simulink model "ver1_mck_system"  (R2019a)
settings: Solver=FixedStepAuto  StartTime=0.0  StopTime=30  FixedStep=10e-5  RelTol=1e-3
InitFcn:
  | ver1_mck_system_m
values from neighbouring files (symbols this model uses):
  C = [1,0 ... (first row only)    [ver1_mck_system_m.m]    (also in ver2_vanderpol_system_m.m)
  dt = 0.001    [ver1_mck_system_m.m]    (also in ver2_vanderpol_system_m.m)
  general_constants = [m ... (first row only)    [ver1_mck_system_m.m]    (also in ver2_vanderpol_system_m.m = [mu])
  H = [1, 0 ... (first row only)    [ver1_mck_system_m.m]    (also in ver2_vanderpol_system_m.m)
  init_cond_cont = [0 ... (first row only)    [ver1_mck_system_m.m]    (also in ver2_vanderpol_system_m.m = [2)
  init_cond_disc = init_cond_cont    [ver1_mck_system_m.m]    (also in ver2_vanderpol_system_m.m)
  MNV = MNstd*MNstd    (= 0.0016)    [ver1_mck_system_m.m]    (also in ver2_vanderpol_system_m.m)
  P_init_disc = MNV*eye(2)    [ver1_mck_system_m.m]    (also in ver2_vanderpol_system_m.m)
  Q = 0*eye(2)*PNV    [ver1_mck_system_m.m]    (also in ver2_vanderpol_system_m.m = 0.2*eye(2)*PNV)
  R = 0.001*eye(2)*MNV    [ver1_mck_system_m.m]    (also in ver2_vanderpol_system_m.m = 60*eye(2)*MNV)
settings Model: Creator=Mehmet  LastModifiedBy=Mehmet

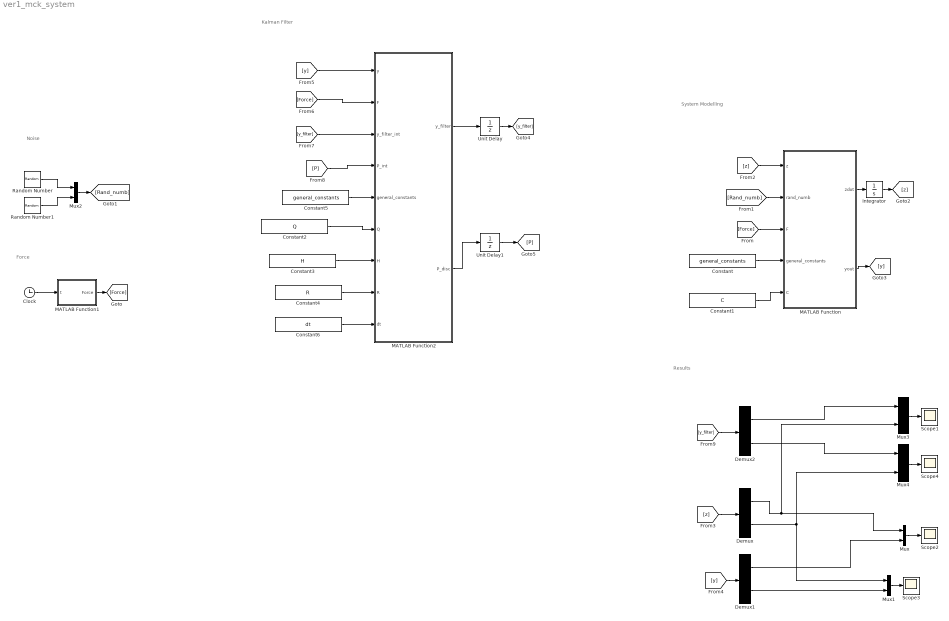
== system ver1_mck_system ==
  note: Noise
  note: Force
  note: Kalman Filter
  note: System Modelling
  note: Results
  Clock : Clock
  Constant : Constant  Value=general_constants  VectorParams1D=off
  Constant1 : Constant  Value=C  VectorParams1D=off
  Constant2 : Constant  Value=Q  VectorParams1D=off
  Constant3 : Constant  Value=H  VectorParams1D=off
  Constant4 : Constant  Value=R  VectorParams1D=off
  Constant5 : Constant  Value=general_constants  VectorParams1D=off
  Constant6 : Constant  Value=dt  VectorParams1D=off
  Demux : Demux  Outputs=2
  Demux1 : Demux  Outputs=2
  Demux2 : Demux  Outputs=2
  Integrator : Integrator  InitialCondition=init_cond_cont
  MATLAB Function : MATLAB Function  TreatAsAtomicUnit=on
  MATLAB Function1 : MATLAB Function  TreatAsAtomicUnit=on
  MATLAB Function2 : MATLAB Function  TreatAsAtomicUnit=on
  Mux{,1..4} (5 alike) : Mux  Inputs=2
  Random Number : RandomNumber  Variance=MNV  SampleTime=dt
  Random Number1 : RandomNumber  Variance=MNV  Seed=5  SampleTime=dt
  Scope{1..4} (4 alike) : Scope
  Unit Delay : UnitDelay  InitialCondition=init_cond_disc  SampleTime=dt  HasFrameUpgradeWarning=on
  Unit Delay1 : UnitDelay  InitialCondition=P_init_disc  SampleTime=dt  HasFrameUpgradeWarning=on
  wires:
  MATLAB Function/1(zdot) -> Integrator/1
  Clock/1 -> MATLAB Function1/1(t)
  Demux/1 -> Mux3/2, Mux/1
  Demux/2 -> Mux1/1, Mux4/2
  Mux/1 -> Scope2/1
  Mux1/1 -> Scope3/1
  Random Number/1 -> Mux2/1
  Random Number1/1 -> Mux2/2
  Demux1/1 -> Mux/2
  Demux1/2 -> Mux1/2
  MATLAB Function1/1(Force) -> [Force]
  [Force] -> MATLAB Function/3(F)
  Mux2/1 -> [Rand_numb]
  [Rand_numb] -> MATLAB Function/2(rand_numb)
  Integrator/1 -> [z]
  [z] -> MATLAB Function/1(z)
  [z] -> Demux/1
  MATLAB Function/2(yout) -> [y]
  [y] -> Demux1/1
  [y] -> MATLAB Function2/1(y)
  [Force] -> MATLAB Function2/2(F)
  MATLAB Function2/1(y_filter) -> Unit Delay/1
  MATLAB Function2/2(P_disc) -> Unit Delay1/1
  Constant/1 -> MATLAB Function/4(general_constants)
  Constant1/1 -> MATLAB Function/5(C)
  Constant2/1 -> MATLAB Function2/6(Q)
  Constant3/1 -> MATLAB Function2/7(H)
  Constant4/1 -> MATLAB Function2/8(R)
  Constant5/1 -> MATLAB Function2/5(general_constants)
  Unit Delay/1 -> [y_filter]
  [y_filter] -> MATLAB Function2/3(y_filter_int)
  Unit Delay1/1 -> [P]
  [P] -> MATLAB Function2/4(P_int)
  Constant6/1 -> MATLAB Function2/9(dt)
  [y_filter] -> Demux2/1
  Mux3/1 -> Scope1/1
  Mux4/1 -> Scope4/1
  Demux2/1 -> Mux3/1
  Demux2/2 -> Mux4/1

== matlab function ver1_mck_system/MATLAB Function1 ==
  data: t input; Force output
function Force = fcn(t)



force_int = cos(2*t);


%% output
Force = force_int;

end

== matlab function ver1_mck_system/MATLAB Function ==
  data: z input; rand_numb input; zdot output; F input; yout output; general_constants input; C input
function [zdot,yout]= fcn(z,rand_numb,F,general_constants,C)

%% constants

m = general_constants(1,1);
c = general_constants(2,1);
k = general_constants(3,1);


%% matrices

A = [0,    1;
    -k/m, -c/m];

B = [0;
    1/m];

%% output
zdot = A*z + B*F;

yout = C*z + rand_numb;

end

== matlab function ver1_mck_system/MATLAB Function2 ==
  data: y input; y_filter output; F input; P_disc output; y_filter_int input; P_int input; general_constants input; Q input; H input; R input; dt input
function [y_filter,P_disc]= fcn(y,F,y_filter_int,P_int,general_constants,Q,H,R,dt)


%% constants

m = general_constants(1,1);
c = general_constants(2,1);
k = general_constants(3,1);


%% System matrices
Atr = [1,          dt;
       -k*dt/m,    (1 - dt*c/m)];
   
Btr = [0;
       dt/m];


%% kalman gain

z_disc = Atr*y_filter_int + Btr*F;
P_disc_int = Atr * P_int * Atr' + Q;
% Compute Kalman gain factor:
K = P_disc_int * H' * inv(H * P_disc_int * H' + R);
% Correction based on observation:

y_filter = z_disc + K*(y - H*z_disc);
P_disc = P_int - K*H*P_int;

%% output

end
